simulink model "vsg"  (R2023b)
settings: Solver=VariableStepAuto  StartTime=0.0  StopTime=1  RelTol=1e-3
InitFcn:
  | Pref = 100;
  | Uref = 24*1.414;
libraries: spsSeriesRLCBranchLib x6, spsCurrentMeasurementLib x2, spsVoltageMeasurementLib x2, spsDCVoltageSourceLib x1, powerlib_extras x1, spsTHDLib x1, spsUniversalBridgeLib x1, sps_lib x1, simulink x1
settings Model: SimulationMode=accelerator  Creator=45276  LastModifiedBy=45276

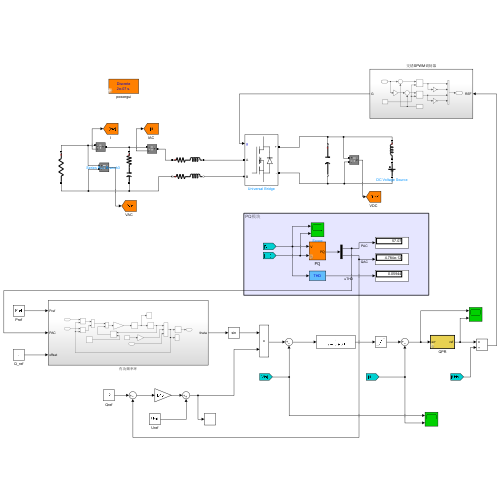
[thumbnail: Simulink's stored preview of the top-level diagram]
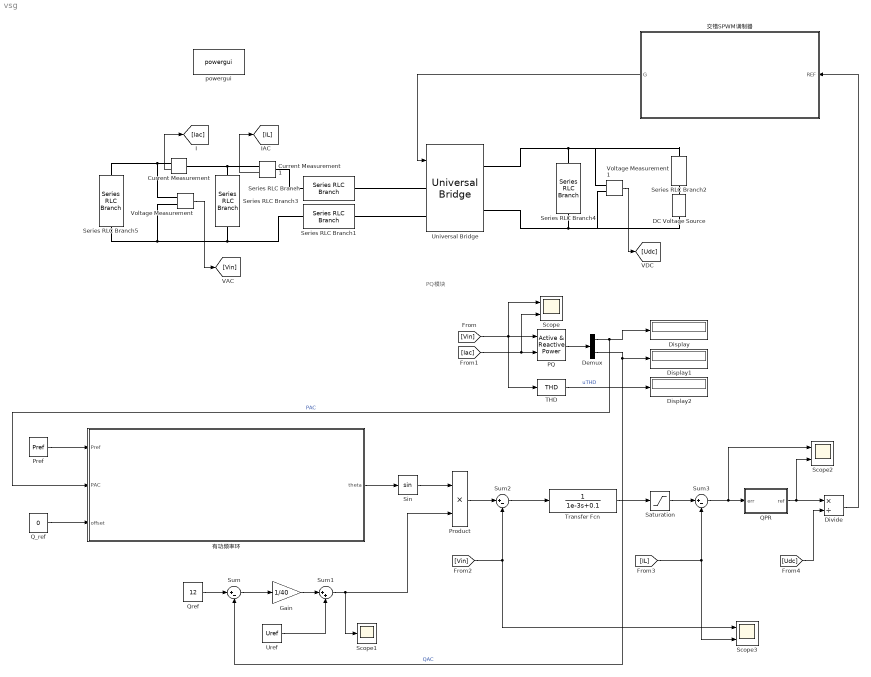
== system vsg ==
  note: PQ模块
  Current Measurement : spsCurrentMeasurementLib/Current Measurement  PhasorSimulation=off  OutputType=Complex  PSBequivalent=0
  Current Measurement1 : spsCurrentMeasurementLib/Current Measurement  PhasorSimulation=off  OutputType=Complex  PSBequivalent=0
  DC Voltage Source : spsDCVoltageSourceLib/DC Voltage Source  Amplitude=45  Measurements=None
  Demux : Demux  Outputs=2
  Display : Display
  Display1 : Display
  Display2 : Display
  Divide : Product  Inputs=*/
  Gain : Gain  Gain=1/40
  PQ : powerlib_extras/Measurements/Active & Reactive Power  f1=50
  Pref : Constant  Value=Pref
  Product : Product
  QPR : Subsystem  TreatAsAtomicUnit=on  mask{Kp=4, Kr=100, Wc=5, Upper=100, Lower=-100}
  Q_ref : Constant  Value=0
  Qref : Constant  Value=12
  Saturation : Saturate  UpperLimit=30  LowerLimit=-30
  Scope : Scope  NumInputPorts=2
  Scope1 : Scope
  Scope2 : Scope  NumInputPorts=2
  Scope3 : Scope  NumInputPorts=2
  Series RLC Branch : spsSeriesRLCBranchLib/Series RLC Branch  LConnTagsString=__new0  RConnTagsString=__new0  BranchType=RL  Resistance=81e-3  Inductance=5e-4  SetiL0=off  InitialCurrent=0  Capacitance=1e-6  Setx0=off  InitialVoltage=0  Measurements=None
  Series RLC Branch1 : spsSeriesRLCBranchLib/Series RLC Branch  LConnTagsString=__new0  RConnTagsString=__new0  BranchType=RL  Resistance=81e-3  Inductance=5e-4  SetiL0=off  InitialCurrent=0  Capacitance=1e-6  Setx0=off  InitialVoltage=0  Measurements=None
  Series RLC Branch2 : spsSeriesRLCBranchLib/Series RLC Branch  LConnTagsString=__new0  RConnTagsString=__new0  BranchType=L  Resistance=1  Inductance=0.05  SetiL0=off  InitialCurrent=0  Capacitance=1e-6  Setx0=off  InitialVoltage=0  Measurements=None
  Series RLC Branch3 : spsSeriesRLCBranchLib/Series RLC Branch  LConnTagsString=__new0  RConnTagsString=__new0  BranchType=RC  Resistance=1  Inductance=1e-3  SetiL0=off  InitialCurrent=0  Capacitance=3e-6  Setx0=off  InitialVoltage=0  Measurements=None
  Series RLC Branch4 : spsSeriesRLCBranchLib/Series RLC Branch  LConnTagsString=__new0  RConnTagsString=__new0  BranchType=C  Resistance=1  Inductance=1e-3  SetiL0=off  InitialCurrent=0  Capacitance=4e-3  Setx0=on  InitialVoltage=45  Measurements=None
  Series RLC Branch5 : spsSeriesRLCBranchLib/Series RLC Branch  LConnTagsString=__new0  RConnTagsString=__new0  BranchType=R  Resistance=10  Inductance=1e-3  SetiL0=off  InitialCurrent=0  Capacitance=1e-6  Setx0=off  InitialVoltage=0  Measurements=None
  Sin : Trigonometry
  Sum : Sum  Inputs=|+-
  Sum1 : Sum  Inputs=|++
  Sum2 : Sum  Inputs=|+-
  Sum3 : Sum  Inputs=|+-
  THD : spsTHDLib/THD  Freq=50  Ts=0
  Transfer Fcn : TransferFcn  Denominator=[1e-3 0.1]
  Universal Bridge : spsUniversalBridgeLib/Universal Bridge  Arms=2  SnubberResistance=1e5  SnubberCapacitance=inf  Device=MOSFET / Diodes  Ron=1e-2  Lon=0  ForwardVoltages="[  0  0  ]"  ForwardVoltage=0  GTOparameters=[ 10e-6 , 20e-6 ]  IGBTparameters=[ 1e-6 , 2e-6 ]  Measurements=None  Measurements_2=None  converterType=Rectifier
  Uref : Constant  Value=Uref
  Voltage Measurement : spsVoltageMeasurementLib/Voltage Measurement  PhasorSimulation=off  OutputType=Complex  PSBequivalent=0
  Voltage Measurement1 : spsVoltageMeasurementLib/Voltage Measurement  PhasorSimulation=off  OutputType=Complex  PSBequivalent=0
  powergui : sps_lib/powergui  Priority=1  SimulationMode=Discrete  SampleTime=2e-07  frequency=60  Iterations=50  frequencyindice=0  Pbase=100e6  ErrMax=1e-4  UnitsV=kV  UnitsW=MW  buscounter=0  FunctionMessages=off  echomessages=off  EnableUseOfTLC=off  CurrentSourceSwitches=off  DisableSnubberDevices=off  DisableRonSwitches=off  DisableVfSwitches=off  DisplayEquations=off  AutomaticDiscreteSolvers=off  SolverType=Tustin/Backward Euler (TBE)  Interpol=off  ExternalGateDelay=off  methode=off  Ts=100  x0status=blocks  SPID=on  SwTol=0  HookPort=off  NonlinearTolerance=1e-4  nMaxIteration=100  ContinueOnMaxIteration=off  RestoreLinks=warning  ResistiveCurrentMeasurement=off  Frange=[0:2:500]  Ylog=off  Xlog=on  ShowGrid=off  save=off  variable=ZData  structure=0  ZoomFFT=off  StartTime=0.0  cycles=1  DisplayStyle=1  fundamental=60  FreqAxis=off  MaxFrequency=1000  frequencyindicesteady=1  RmsSteady=1  display=off
  交错SPWM调制器 : Subsystem
  有功频率环 : Subsystem
  wires:
  Voltage Measurement/1 -> [Vin]
  Current Measurement/1 -> [Iac]
  Current Measurement1/1 -> [IL]
  Voltage Measurement1/1 -> [Udc]
  [Vin] -> Scope/1, THD/1, PQ/1
  [Iac] -> Scope/2, PQ/2
  PQ/1 -> Demux/1
  Demux/1 -> 有功频率环/2(PAC), Display/1  "PAC"
  Demux/2 -> Display1/1, Sum/2  "QAC"
  THD/1 -> Display2/1  "uTHD"
  Pref/1 -> 有功频率环/1(Pref)
  Q_ref/1 -> 有功频率环/3(offset)
  Qref/1 -> Sum/1
  Sum/1 -> Gain/1
  Gain/1 -> Sum1/1
  Uref/1 -> Sum1/2
  有功频率环/1(theta) -> Sin/1
  Sin/1 -> Product/1
  Sum1/1 -> Scope1/1, Product/2
  Product/1 -> Sum2/1
  [Vin] -> Sum2/2, Scope3/1
  Sum2/1 -> Transfer Fcn/1
  Transfer Fcn/1 -> Saturation/1
  Saturation/1 -> Sum3/1
  QPR/1(ref) -> Scope2/2, Divide/1
  [Udc] -> Divide/2
  Divide/1 -> 交错SPWM调制器/1(REF)
  交错SPWM调制器/1(G) -> Universal Bridge/1
  Sum3/1 -> Scope2/1, QPR/1(err)
  [IL] -> Scope3/2, Sum3/2
  connections:
  Series RLC Branch/RConn1 -- Universal Bridge/LConn1
  Series RLC Branch1/RConn1 -- Universal Bridge/LConn2
  Series RLC Branch1/LConn1 -- Series RLC Branch3/RConn1 -- Voltage Measurement/LConn2 -- Series RLC Branch5/RConn1
  Universal Bridge/RConn1 -- Series RLC Branch2/LConn1 -- Voltage Measurement1/LConn1 -- Series RLC Branch4/LConn1
  Universal Bridge/RConn2 -- DC Voltage Source/LConn1 -- Voltage Measurement1/LConn2 -- Series RLC Branch4/RConn1
  Voltage Measurement/LConn1 -- Series RLC Branch5/LConn1 -- Current Measurement/RConn1
  Current Measurement/LConn1 -- Current Measurement1/RConn1 -- Series RLC Branch3/LConn1
  Current Measurement1/LConn1 -- Series RLC Branch/LConn1
  DC Voltage Source/RConn1 -- Series RLC Branch2/RConn1

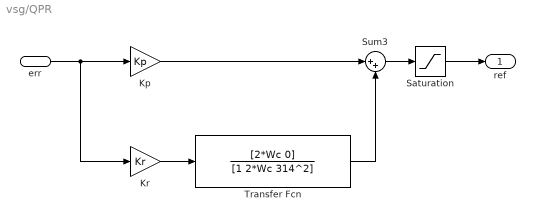
== system vsg/QPR ==
  err : Inport
  Kp : Gain  Gain=Kp
  Kr : Gain  Gain=Kr
  Saturation : Saturate  UpperLimit=Upper  LowerLimit=Lower
  Sum3 : Sum  Inputs=|++
  Transfer Fcn : TransferFcn  Numerator=[2*Wc 0]  Denominator=[1 2*Wc 314^2]
  ref : Outport
  wires:
  Saturation/1 -> ref/1
  Transfer Fcn/1 -> Sum3/2
  Kr/1 -> Transfer Fcn/1
  err/1 -> Kp/1, Kr/1
  Sum3/1 -> Saturation/1
  Kp/1 -> Sum3/1

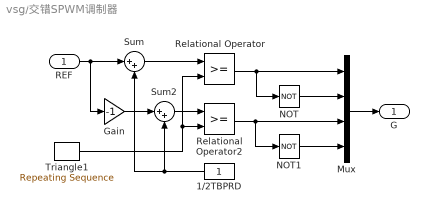
== system vsg/交错SPWM调制器 ==
  REF : Inport
  1/2TBPRD : Constant
  Gain : Gain  Gain=-1
  Mux : Mux
  NOT : Logic  Operator=NOT  IconShape=distinctive  AllPortsSameDT=off  OutDataTypeStr=boolean
  NOT1 : Logic  Operator=NOT  IconShape=distinctive  AllPortsSameDT=off  OutDataTypeStr=boolean
  Relational Operator : RelationalOperator  OutDataTypeStr=boolean  InputSameDT=off
  Relational Operator2 : RelationalOperator  OutDataTypeStr=boolean  InputSameDT=off
  Sum : Sum  Inputs=|++
  Sum2 : Sum  Inputs=|++
  Triangle1 : simulink/Sources/Repeating Sequence  rep_seq_t=[0 1/16000/2 1/16000]  rep_seq_y=[0 2 0]
  G : Outport
  wires:
  Relational Operator2/1 -> Mux/3, NOT1/1
  NOT1/1 -> Mux/4
  Mux/1 -> G/1
  NOT/1 -> Mux/2
  Relational Operator/1 -> Mux/1, NOT/1
  1/2TBPRD/1 -> Sum2/2, Sum/2
  Sum2/1 -> Relational Operator2/1
  Gain/1 -> Sum2/1
  REF/1 -> Sum/1, Gain/1
  Sum/1 -> Relational Operator/1
  Triangle1/1 -> Relational Operator/2, Relational Operator2/2

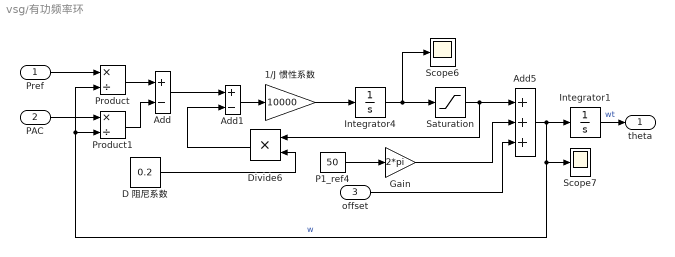
== system vsg/有功频率环 ==
  Pref : Inport
  PAC : Inport  Port=2
  offset : Inport  Port=3
  1/J 惯性系数 : Gain  Gain=10000
  Add : Sum  Inputs=+-
  Add1 : Sum  Inputs=+-
  Add5 : Sum  Inputs=+++
  D 阻尼系数 : Constant  Value=0.2
  Divide6 : Product  Inputs=**
  Gain : Gain  Gain=2*pi
  Integrator1 : Integrator  WrapState=on  WrappedStateUpperValue=2*pi  WrappedStateLowerValue=0
  Integrator4 : Integrator
  P1_ref4 : Constant  Value=50
  Product : Product  Inputs=*/
  Product1 : Product  Inputs=*/
  Saturation : Saturate  UpperLimit=15  LowerLimit=-10
  Scope6 : Scope
  Scope7 : Scope
  theta : Outport
  wires:
  Integrator4/1 -> Scope6/1, Saturation/1
  Integrator1/1 -> theta/1  "wt"
  Saturation/1 -> Add5/1, Divide6/1
  Add5/1 -> Integrator1/1, Scope7/1, Product/2, Product1/2  "w"
  Product1/1 -> Add/2
  Product/1 -> Add/1
  1/J 惯性系数/1 -> Integrator4/1
  Gain/1 -> Add5/2
  PAC/1 -> Product1/1
  Pref/1 -> Product/1
  Divide6/1 -> Add1/2
  D 阻尼系数/1 -> Divide6/2
  Add/1 -> Add1/1
  P1_ref4/1 -> Gain/1
  offset/1 -> Add5/3
  Add1/1 -> 1/J 惯性系数/1
